simulink model "L400_airframe"  (R2024b)
settings: Solver=FixedStepAuto  StartTime=0  StopTime=20  FixedStep=5/1000  RelTol=1e-3
model workspace (MAT data in the model file):
  Sig : Simulink.Signal (value not decoded)
  Sig1 : Simulink.Signal (value not decoded)
  Sig2 : Simulink.Signal (value not decoded)
  Sig3 : Simulink.Signal (value not decoded)
  Sig4 : Simulink.Signal (value not decoded)
  Sig5 : Simulink.Signal (value not decoded)
  Sig6 : Simulink.Signal (value not decoded)
undefined symbols (not defined in the file or in its folder): convertTo, datetime, db, Earth, F, lambda, Light, MIL, WGS84, WMM2020
libraries: aerolibconvert2 x18, aerolibasang x5, aerolibtransform2 x3, aerolibwind2 x3, aerolibactuator x2, matrix_library x2, shared6dof x1, aerolibatmos2 x1, aerolibgravity2 x1
(part 4 of 4)

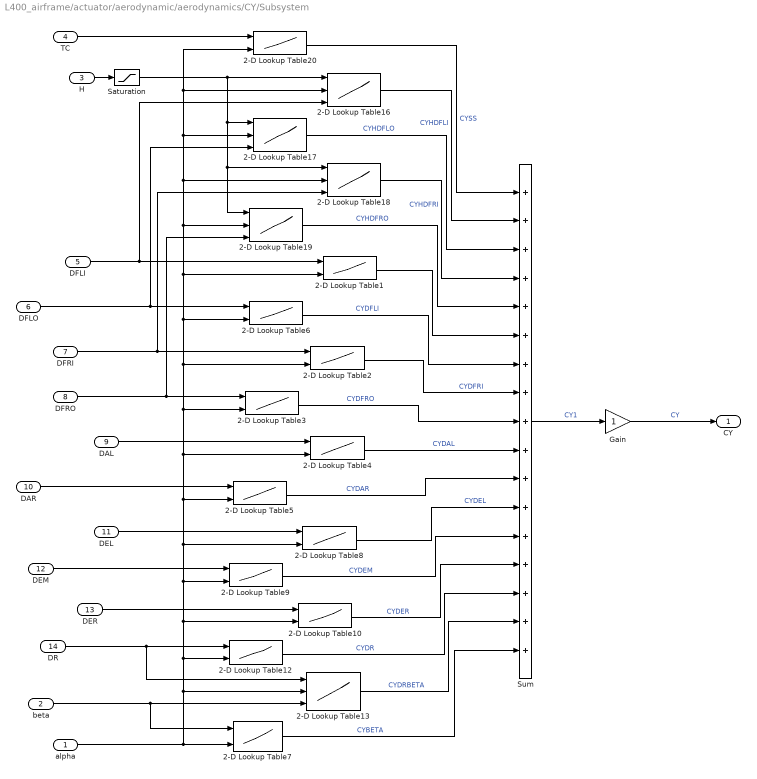
== system L400_airframe/actuator/aerodynamic/aerodynamics/CY/Subsystem ==
  alpha : Inport  Unit=deg
  beta : Inport  Port=2  Unit=deg
  H : Inport  Port=3
  TC : Inport  Port=4
  DFLI : Inport  Port=5
  DFLO : Inport  Port=6
  DFRI : Inport  Port=7
  DFRO : Inport  Port=8
  DAL : Inport  Port=9
  DAR : Inport  Port=10
  DEL : Inport  Port=11
  DEM : Inport  Port=12
  DER : Inport  Port=13
  DR : Inport  Port=14
  2-D Lookup Table1 : Lookup_n-D  LookupTableObject=''  BreakpointsForDimension1=db.aerody.VDF  BreakpointsForDimension2=db.aerody.VALPHA  BreakpointsForDimension1FirstPoint=10  BreakpointsForDimension2FirstPoint=10  BreakpointsForDimension1Spacing=12  BreakpointsForDimension2Spacing=12  IndexSearchMethod=Linear search  BeginIndexSearchUsingPreviousIndexResult=on  Table=db.aerody.CYDFLI  ExtrapMethod=Clip  DiagnosticForOutOfRangeInput=Warning  InternalRulePriority=Speed  RndMeth=Simplest
      settings: InputPortMap=u0,u1
  2-D Lookup Table10 : Lookup_n-D  LookupTableObject=''  BreakpointsForDimension1=db.aerody.VDE  BreakpointsForDimension2=db.aerody.VALPHA  BreakpointsForDimension1FirstPoint=10  BreakpointsForDimension2FirstPoint=10  BreakpointsForDimension1Spacing=12  BreakpointsForDimension2Spacing=12  IndexSearchMethod=Linear search  BeginIndexSearchUsingPreviousIndexResult=on  Table=db.aerody.CYDER  ExtrapMethod=Clip  DiagnosticForOutOfRangeInput=Warning  InternalRulePriority=Speed  RndMeth=Simplest
      settings: InputPortMap=u0,u1
  2-D Lookup Table12 : Lookup_n-D  LookupTableObject=''  BreakpointsForDimension1=db.aerody.VDR  BreakpointsForDimension2=db.aerody.VALPHA  BreakpointsForDimension1FirstPoint=10  BreakpointsForDimension2FirstPoint=10  BreakpointsForDimension1Spacing=12  BreakpointsForDimension2Spacing=12  IndexSearchMethod=Linear search  BeginIndexSearchUsingPreviousIndexResult=on  Table=db.aerody.CYDR  ExtrapMethod=Clip  DiagnosticForOutOfRangeInput=Warning  InternalRulePriority=Speed  RndMeth=Simplest
      settings: InputPortMap=u0,u1
  2-D Lookup Table13 : Lookup_n-D  NumberOfTableDimensions=3  LookupTableObject=''  BreakpointsForDimension1=db.aerody.VDR  BreakpointsForDimension2=db.aerody.VALPHA  BreakpointsForDimension3=db.aerody.VBETA  BreakpointsForDimension1FirstPoint=10  BreakpointsForDimension2FirstPoint=10  BreakpointsForDimension1Spacing=12  BreakpointsForDimension2Spacing=12  IndexSearchMethod=Linear search  BeginIndexSearchUsingPreviousIndexResult=on  Table=db.aerody.CYDRBETA  ExtrapMethod=Clip  DiagnosticForOutOfRangeInput=Warning  InternalRulePriority=Speed  RndMeth=Simplest
      settings: InputPortMap=u0,u1,u2
  2-D Lookup Table16 : Lookup_n-D  NumberOfTableDimensions=3  LookupTableObject=''  BreakpointsForDimension1=db.aerody.VH  BreakpointsForDimension2=db.aerody.VALPHA  BreakpointsForDimension3=db.aerody.VDF  BreakpointsForDimension1FirstPoint=10  BreakpointsForDimension2FirstPoint=10  BreakpointsForDimension1Spacing=12  BreakpointsForDimension2Spacing=12  IndexSearchMethod=Linear search  BeginIndexSearchUsingPreviousIndexResult=on  Table=db.aerody.CYHDFLI  ExtrapMethod=Clip  DiagnosticForOutOfRangeInput=Warning  InternalRulePriority=Speed  RndMeth=Simplest
      settings: InputPortMap=u0,u1,u2
  2-D Lookup Table17 : Lookup_n-D  NumberOfTableDimensions=3  LookupTableObject=''  BreakpointsForDimension1=db.aerody.VH  BreakpointsForDimension2=db.aerody.VALPHA  BreakpointsForDimension3=db.aerody.VDF  BreakpointsForDimension1FirstPoint=10  BreakpointsForDimension2FirstPoint=10  BreakpointsForDimension1Spacing=12  BreakpointsForDimension2Spacing=12  IndexSearchMethod=Linear search  BeginIndexSearchUsingPreviousIndexResult=on  Table=db.aerody.CYHDFLO  ExtrapMethod=Clip  DiagnosticForOutOfRangeInput=Warning  InternalRulePriority=Speed  RndMeth=Simplest
      settings: InputPortMap=u0,u1,u2
  2-D Lookup Table18 : Lookup_n-D  NumberOfTableDimensions=3  LookupTableObject=''  BreakpointsForDimension1=db.aerody.VH  BreakpointsForDimension2=db.aerody.VALPHA  BreakpointsForDimension3=db.aerody.VDF  BreakpointsForDimension1FirstPoint=10  BreakpointsForDimension2FirstPoint=10  BreakpointsForDimension1Spacing=12  BreakpointsForDimension2Spacing=12  IndexSearchMethod=Linear search  BeginIndexSearchUsingPreviousIndexResult=on  Table=db.aerody.CYHDFRI  ExtrapMethod=Clip  DiagnosticForOutOfRangeInput=Warning  InternalRulePriority=Speed  RndMeth=Simplest
      settings: InputPortMap=u0,u1,u2
  2-D Lookup Table19 : Lookup_n-D  NumberOfTableDimensions=3  LookupTableObject=''  BreakpointsForDimension1=db.aerody.VH  BreakpointsForDimension2=db.aerody.VALPHA  BreakpointsForDimension3=db.aerody.VDF  BreakpointsForDimension1FirstPoint=10  BreakpointsForDimension2FirstPoint=10  BreakpointsForDimension1Spacing=12  BreakpointsForDimension2Spacing=12  IndexSearchMethod=Linear search  BeginIndexSearchUsingPreviousIndexResult=on  Table=db.aerody.CYHDFRO  ExtrapMethod=Clip  DiagnosticForOutOfRangeInput=Warning  InternalRulePriority=Speed  RndMeth=Simplest
      settings: InputPortMap=u0,u1,u2
  2-D Lookup Table2 : Lookup_n-D  LookupTableObject=''  BreakpointsForDimension1=db.aerody.VDF  BreakpointsForDimension2=db.aerody.VALPHA  BreakpointsForDimension1FirstPoint=10  BreakpointsForDimension2FirstPoint=10  BreakpointsForDimension1Spacing=12  BreakpointsForDimension2Spacing=12  IndexSearchMethod=Linear search  BeginIndexSearchUsingPreviousIndexResult=on  Table=db.aerody.CYDFRI  ExtrapMethod=Clip  DiagnosticForOutOfRangeInput=Warning  InternalRulePriority=Speed  RndMeth=Simplest
      settings: InputPortMap=u0,u1
  2-D Lookup Table20 : Lookup_n-D  LookupTableObject=''  BreakpointsForDimension1=db.aerody.VTC  BreakpointsForDimension2=db.aerody.VALPHA  BreakpointsForDimension1FirstPoint=10  BreakpointsForDimension2FirstPoint=10  BreakpointsForDimension1Spacing=12  BreakpointsForDimension2Spacing=12  IndexSearchMethod=Linear search  BeginIndexSearchUsingPreviousIndexResult=on  Table=db.aerody.CYSS  ExtrapMethod=Clip  DiagnosticForOutOfRangeInput=Warning  InternalRulePriority=Speed  RndMeth=Simplest
      settings: InputPortMap=u0,u1
  2-D Lookup Table3 : Lookup_n-D  LookupTableObject=''  BreakpointsForDimension1=db.aerody.VDF  BreakpointsForDimension2=db.aerody.VALPHA  BreakpointsForDimension1FirstPoint=10  BreakpointsForDimension2FirstPoint=10  BreakpointsForDimension1Spacing=12  BreakpointsForDimension2Spacing=12  IndexSearchMethod=Linear search  BeginIndexSearchUsingPreviousIndexResult=on  Table=db.aerody.CYDFRO  ExtrapMethod=Clip  DiagnosticForOutOfRangeInput=Warning  InternalRulePriority=Speed  RndMeth=Simplest
      settings: InputPortMap=u0,u1
  2-D Lookup Table4 : Lookup_n-D  LookupTableObject=''  BreakpointsForDimension1=db.aerody.VDA  BreakpointsForDimension2=db.aerody.VALPHA  BreakpointsForDimension1FirstPoint=10  BreakpointsForDimension2FirstPoint=10  BreakpointsForDimension1Spacing=12  BreakpointsForDimension2Spacing=12  IndexSearchMethod=Linear search  BeginIndexSearchUsingPreviousIndexResult=on  Table=db.aerody.CYDAL  ExtrapMethod=Clip  DiagnosticForOutOfRangeInput=Warning  InternalRulePriority=Speed  RndMeth=Simplest
      settings: InputPortMap=u0,u1
  2-D Lookup Table5 : Lookup_n-D  LookupTableObject=''  BreakpointsForDimension1=db.aerody.VDA  BreakpointsForDimension2=db.aerody.VALPHA  BreakpointsForDimension1FirstPoint=10  BreakpointsForDimension2FirstPoint=10  BreakpointsForDimension1Spacing=12  BreakpointsForDimension2Spacing=12  IndexSearchMethod=Linear search  BeginIndexSearchUsingPreviousIndexResult=on  Table=db.aerody.CYDAR  ExtrapMethod=Clip  DiagnosticForOutOfRangeInput=Warning  InternalRulePriority=Speed  RndMeth=Simplest
      settings: InputPortMap=u0,u1
  2-D Lookup Table6 : Lookup_n-D  LookupTableObject=''  BreakpointsForDimension1=db.aerody.VDF  BreakpointsForDimension2=db.aerody.VALPHA  BreakpointsForDimension1FirstPoint=10  BreakpointsForDimension2FirstPoint=10  BreakpointsForDimension1Spacing=12  BreakpointsForDimension2Spacing=12  IndexSearchMethod=Linear search  BeginIndexSearchUsingPreviousIndexResult=on  Table=db.aerody.CYDFLO  ExtrapMethod=Clip  DiagnosticForOutOfRangeInput=Warning  InternalRulePriority=Speed  RndMeth=Simplest
      settings: InputPortMap=u0,u1
  2-D Lookup Table7 : Lookup_n-D  LookupTableObject=''  BreakpointsForDimension1=db.aerody.VBETA  BreakpointsForDimension2=db.aerody.VALPHA  BreakpointsForDimension1FirstPoint=10  BreakpointsForDimension2FirstPoint=10  BreakpointsForDimension1Spacing=12  BreakpointsForDimension2Spacing=12  IndexSearchMethod=Linear search  BeginIndexSearchUsingPreviousIndexResult=on  Table=db.aerody.CYBETA  ExtrapMethod=Clip  DiagnosticForOutOfRangeInput=Warning  InternalRulePriority=Speed  RndMeth=Simplest
      settings: InputPortMap=u0,u1
  2-D Lookup Table8 : Lookup_n-D  LookupTableObject=''  BreakpointsForDimension1=db.aerody.VDE  BreakpointsForDimension2=db.aerody.VALPHA  BreakpointsForDimension1FirstPoint=10  BreakpointsForDimension2FirstPoint=10  BreakpointsForDimension1Spacing=12  BreakpointsForDimension2Spacing=12  IndexSearchMethod=Linear search  BeginIndexSearchUsingPreviousIndexResult=on  Table=db.aerody.CYDEL  ExtrapMethod=Clip  DiagnosticForOutOfRangeInput=Warning  InternalRulePriority=Speed  RndMeth=Simplest
      settings: InputPortMap=u0,u1
  2-D Lookup Table9 : Lookup_n-D  LookupTableObject=''  BreakpointsForDimension1=db.aerody.VDE  BreakpointsForDimension2=db.aerody.VALPHA  BreakpointsForDimension1FirstPoint=10  BreakpointsForDimension2FirstPoint=10  BreakpointsForDimension1Spacing=12  BreakpointsForDimension2Spacing=12  IndexSearchMethod=Linear search  BeginIndexSearchUsingPreviousIndexResult=on  Table=db.aerody.CYDEM  ExtrapMethod=Clip  DiagnosticForOutOfRangeInput=Warning  InternalRulePriority=Speed  RndMeth=Simplest
      settings: InputPortMap=u0,u1
  Gain : Gain
  Saturation : Saturate  UpperLimit=5.8  LowerLimit=0
  Sum : Sum  Inputs=17
  CY : Outport
  wires:
  2-D Lookup Table17/1 -> Sum/3  "CYHDFLO"
  2-D Lookup Table13/1 -> Sum/16  "CYDRBETA"
  2-D Lookup Table1/1 -> Sum/6
  alpha/1 -> 2-D Lookup Table7/2, 2-D Lookup Table20/2, 2-D Lookup Table16/2, 2-D Lookup Table17/2, 2-D Lookup Table18/2, 2-D Lookup Table19/2, 2-D Lookup Table1/2, 2-D Lookup Table6/2, 2-D Lookup Table2/2, 2-D Lookup Table3/2, 2-D Lookup Table4/2, 2-D Lookup Table5/2, 2-D Lookup Table8/2, 2-D Lookup Table9/2, 2-D Lookup Table10/2, 2-D Lookup Table12/2, 2-D Lookup Table13/2
  beta/1 -> 2-D Lookup Table7/1, 2-D Lookup Table13/3
  2-D Lookup Table20/1 -> Sum/1  "CYSS"
  2-D Lookup Table7/1 -> Sum/17  "CYBETA"
  2-D Lookup Table12/1 -> Sum/15  "CYDR"
  2-D Lookup Table6/1 -> Sum/7  "CYDFLI"
  DFRI/1 -> 2-D Lookup Table18/3, 2-D Lookup Table2/1
  2-D Lookup Table2/1 -> Sum/8  "CYDFRI"
  DFRO/1 -> 2-D Lookup Table19/3, 2-D Lookup Table3/1
  DFLI/1 -> 2-D Lookup Table16/3, 2-D Lookup Table1/1
  2-D Lookup Table9/1 -> Sum/13  "CYDEM"
  2-D Lookup Table16/1 -> Sum/2  "CYHDFLI"
  Sum/1 -> Gain/1  "CY1"
  DFLO/1 -> 2-D Lookup Table6/1, 2-D Lookup Table17/3
  2-D Lookup Table8/1 -> Sum/12  "CYDEL"
  2-D Lookup Table19/1 -> Sum/5  "CYHDFRO"
  Gain/1 -> CY/1  "CY"
  2-D Lookup Table5/1 -> Sum/11  "CYDAR"
  H/1 -> Saturation/1
  2-D Lookup Table10/1 -> Sum/14  "CYDER"
  2-D Lookup Table4/1 -> Sum/10  "CYDAL"
  2-D Lookup Table18/1 -> Sum/4  "CYHDFRI"
  DR/1 -> 2-D Lookup Table12/1, 2-D Lookup Table13/1
  DAL/1 -> 2-D Lookup Table4/1
  2-D Lookup Table3/1 -> Sum/9  "CYDFRO"
  DAR/1 -> 2-D Lookup Table5/1
  DER/1 -> 2-D Lookup Table10/1
  TC/1 -> 2-D Lookup Table20/1
  DEL/1 -> 2-D Lookup Table8/1
  DEM/1 -> 2-D Lookup Table9/1
  Saturation/1 -> 2-D Lookup Table19/1, 2-D Lookup Table18/1, 2-D Lookup Table17/1, 2-D Lookup Table16/1

== matlab function L400_airframe/actuator/landgear/Subsystem/MATLAB Function ==
  data: theta input; y output; varphi input; lambda input; delta input
function y = fcn(theta,varphi,lambda,delta)
y = arctan{(cos(theta)cos(varphi)cos(lambda)-sin(theta)sin(lambda))cos(lambda)+...
    [(sin(theta)cos(lambda)+cos(theta)cos(varphi)sin(lambda))cos(delta)-cos(theta)sin(varphi)sin(delta)]sin(lambda)}/...
    {(cos(theta)cos(varphi)cos(lambda)-sin(theta)sin(lambda))sin(lambda) - ...
    [(sin(theta)cos(lambda)+cos(theta)cos(varphi)sin(lambda))cos(delta)-cos(theta)sin(varphi)sin(delta)]cos(lambda) };
y = u;
